simulink model "EvitaParedes"  (R2023b)
settings: Solver=FixedStepAuto  StartTime=0.0  StopTime=inf  RelTol=1e-3  EnableMultiTasking=on
libraries: simulink x3
settings Model: ExtModeTrigDuration=2  Creator=Usuario  LastModifiedBy=Usuario
settings OptimizationCC: EnhancedBackFolding=on  PassReuseOutputArgsAs=Individual arguments  ZeroExternalMemoryAtStartup=off  ZeroInternalMemoryAtStartup=off  MaxStackSize=64  OptimizeBlockOrder=speed  DifferentSizesBufferReuse=on  OptimizationCustomize=off  EfficientTunableParamExpr=on
settings DebuggingCC: ParameterTunabilityLossMsg=error
settings HardwareCC: ProdBitPerInt=16  ProdBitPerPointer=16  ProdBitPerSizeT=16  ProdBitPerPtrDiffT=16  ProdLargestAtomicFloat=None  ProdWordSize=8  ProdHWDeviceType=Atmel->AVR  UseEmbeddedCoderFeatures=off  UseSimulinkCoderFeatures=off
settings SFSimCC: MATLABDynamicMemAlloc=off
settings RTWCC: Description=Embedded Coder  SystemTargetFile=ert.tlc  HardwareBoard=Arduino Mega 2560  TemplateMakefile=ert_default_tmf  Toolchain=Arduino AVR  BuildConfiguration=Faster Runs
settings CodeAppCC: ForceParamTrailComments=on  IgnoreCustomStorageClasses=off  OperatorAnnotations=on  SimulinkDataObjDesc=on  SFDataObjDesc=on  MangleLength=10  InsertBlockDesc=on
settings ERTTargetCC: SupportContinuousTime=on  SupportNonInlinedSFcns=on  SupportVariableSizeSignals=on  ExtModeTransport=3  ExtModeStaticAlloc=on  ExtModeAutomaticAllocSize=off  ExtModeStaticAllocSize=2048  ExtModeMexFile=ext_xcp  ExtModeIntrfLevel=Level2 - Open

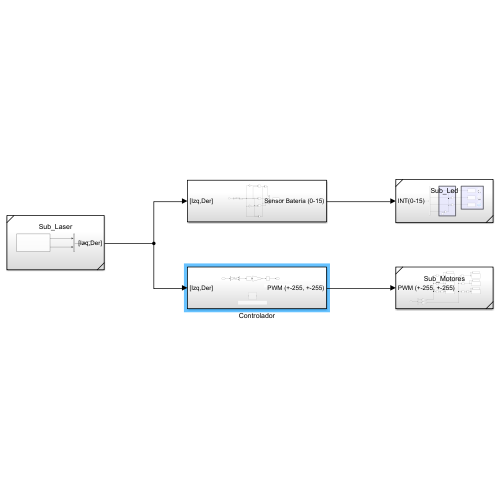
[thumbnail: Simulink's stored preview of the top-level diagram]
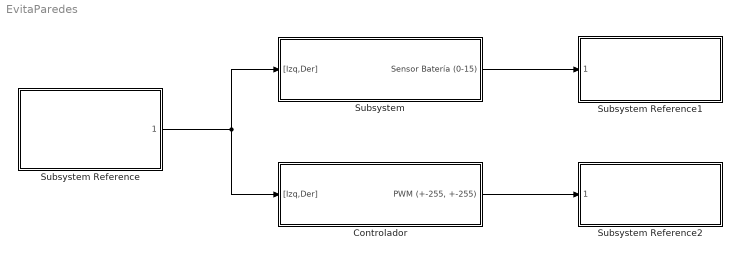
== system EvitaParedes ==
  Controlador : Subsystem
  Subsystem : Subsystem
  Subsystem Reference : Subsystem  ReferencedSubsystem=Sub_Laser
  Subsystem Reference1 : Subsystem  ReferencedSubsystem=Sub_Led
  Subsystem Reference2 : Subsystem  ReferencedSubsystem=Sub_Motores
  wires:
  Controlador/1("PWM (+-255, +-255)") -> Subsystem Reference2/1
  Subsystem Reference/1 -> Controlador/1("[Izq,Der]"), Subsystem/1("[Izq,Der]")
  Subsystem/1(Sensor Batería (0-15)) -> Subsystem Reference1/1

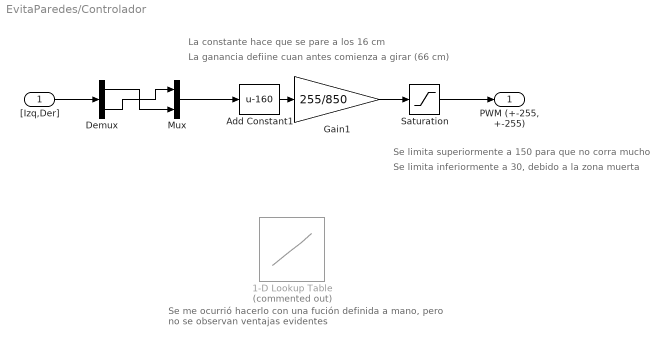
== system EvitaParedes/Controlador ==
  note: Se limita superiormente a 150 para que no corra mucho
  note: Se limita inferiormente a 30, debido a la zona muerta
  note: Se me ocurrió hacerlo con una fución definida a mano, pero no se observan ventajas evidentes
  note: La ganancia defiine cuan antes comienza a girar (66 cm)
  note: La constante hace que se pare a los 16 cm
  "[Izq,Der]" : Inport
  1-D Lookup Table : Lookup_n-D  Commented=on  NumberOfTableDimensions=1  BreakpointsForDimension1=[0;180;220;260;300;400;750;800]  BreakpointsForDimension1DataTypeStr=double  Table=[0;0;5;20;75;90;100;100]  TableDataTypeStr=double  IntermediateResultsDataTypeStr=double  ExtrapMethod=Clip  InternalRulePriority=Speed  OutDataTypeStr=double  RndMeth=Simplest  FractionDataTypeStr=double
  Add Constant1 : Bias  Bias=-160  SaturateOnIntegerOverflow=off
  Demux : Demux  Outputs=2
  Gain1 : Gain  Gain=255/850
  Mux : Mux  Inputs=2
  Saturation : Saturate  UpperLimit=150  LowerLimit=0
  "PWM (+-255, +-255)" : Outport
  wires:
  Demux/1 -> Mux/2
  Mux/1 -> Add Constant1/1
  Saturation/1 -> "PWM (+-255, +-255)"/1
  Demux/2 -> Mux/1
  "[Izq,Der]"/1 -> Demux/1
  Add Constant1/1 -> Gain1/1
  Gain1/1 -> Saturation/1

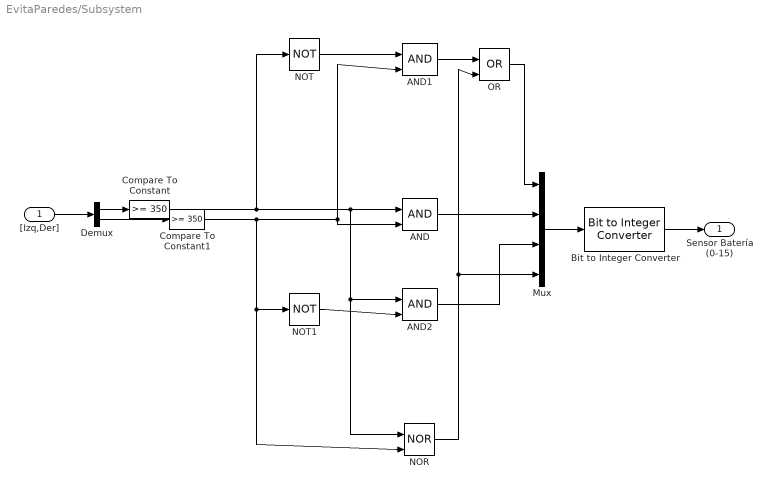
== system EvitaParedes/Subsystem ==
  "[Izq,Der]" : Inport
  AND : Logic  IconShape=distinctive  AllPortsSameDT=off  OutDataTypeStr=boolean
  AND1 : Logic  IconShape=distinctive  AllPortsSameDT=off  OutDataTypeStr=boolean
  AND2 : Logic  IconShape=distinctive  AllPortsSameDT=off  OutDataTypeStr=boolean
  Bit to Integer Converter : simulink/Logic and Bit Operations/Bit to Integer Converter  nbits=4  bitOrder=MSB first  signedOutputValues=Unsigned  outDtype=Inherit via internal rule  outDtypeSigned=Inherit via internal rule
  Compare To Constant : simulink/Logic and Bit Operations/Compare To Constant  relop=>=  const=350  OutDataTypeStr=boolean
  Compare To Constant1 : simulink/Logic and Bit Operations/Compare To Constant  relop=>=  const=350  OutDataTypeStr=boolean
  Demux : Demux  Outputs=2
  Mux : Mux
  NOR : Logic  Operator=NOR  IconShape=distinctive  AllPortsSameDT=off  OutDataTypeStr=boolean
  NOT : Logic  Operator=NOT  IconShape=distinctive  AllPortsSameDT=off  OutDataTypeStr=boolean
  NOT1 : Logic  Operator=NOT  IconShape=distinctive  AllPortsSameDT=off  OutDataTypeStr=boolean
  OR : Logic  Operator=OR  IconShape=distinctive  AllPortsSameDT=off  OutDataTypeStr=boolean
  Sensor Batería (0-15) : Outport
  wires:
  Demux/1 -> Compare To Constant/1
  Demux/2 -> Compare To Constant1/1
  Mux/1 -> Bit to Integer Converter/1
  "[Izq,Der]"/1 -> Demux/1
  Bit to Integer Converter/1 -> Sensor Batería (0-15)/1
  Compare To Constant/1 -> NOT/1, AND/1, NOR/1, AND2/1
  Compare To Constant1/1 -> NOR/2, NOT1/1, AND/2, AND1/2
  OR/1 -> Mux/1
  AND/1 -> Mux/2
  NOT/1 -> AND1/1
  AND1/1 -> OR/1
  NOT1/1 -> AND2/2
  NOR/1 -> Mux/4, OR/2
  AND2/1 -> Mux/3
